simulink model "Quad_F450_Model"  (R2023a)
settings: Solver=FixedStepAuto  StartTime=0.0  StopTime=inf  FixedStep=Copter.SimTs  RelTol=1e-3
InitFcn:
  | load("motor_data.mat")
  | run("Parameters.m")
undefined symbols (not defined in the file or in its folder): Controller, Copter, DiscIntNeverNeededParam, Earth, init, Keyboard, motor_data, w_der_filt, WGS84
libraries: sharedutil x12, slpidlib x8, sharedtransform x5, aerolibpropulsionsys x4, simulink_extras x3, matrix_library x3, shared6dof x1, aerolibtransform2 x1, aerolibatmos2 x1, aerolibsim3d x1, sim3dlib x1
(part 1 of 3)
settings Model: Creator=burak  LastModifiedBy=burak

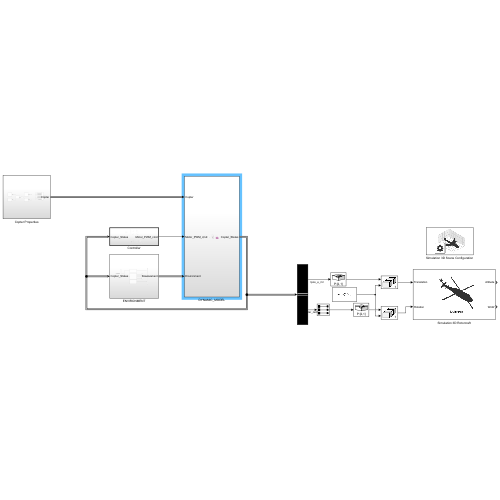
[thumbnail: Simulink's stored preview of the top-level diagram]
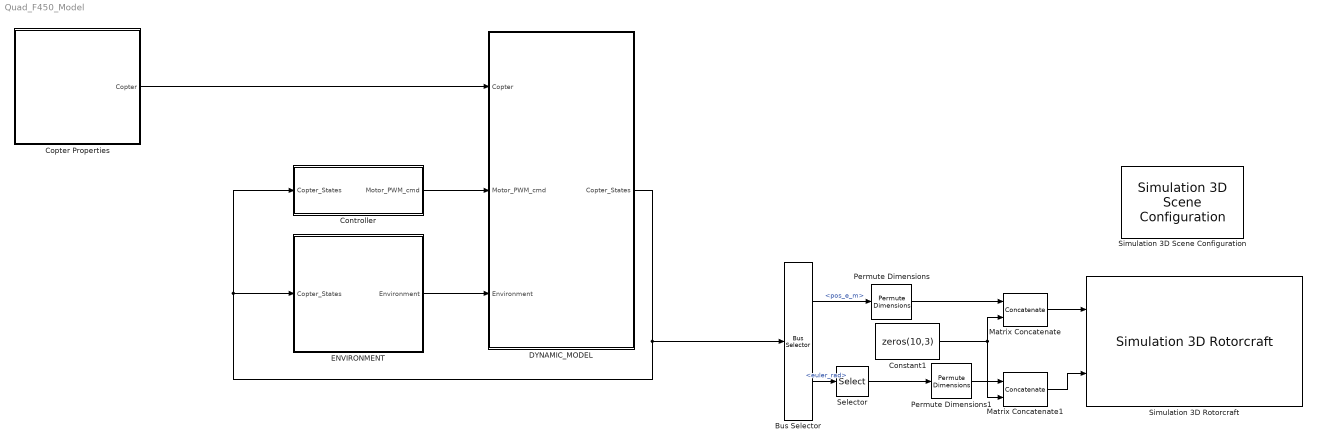
== system Quad_F450_Model ==
  Bus Selector : BusSelector  OutputSignals=pos_e_m,euler_rad
  Constant1 : Constant  Value=zeros(10,3)
  Controller : Subsystem  TreatAsAtomicUnit=on  SystemSampleTime=Controller.Ts
  Copter Properties : Subsystem
  DYNAMIC_MODEL : Subsystem
  ENVIRONMENT : Subsystem
  Matrix Concatenate : Concatenate  Mode=Multidimensional array
  Matrix Concatenate1 : Concatenate  Mode=Multidimensional array
  Permute Dimensions : PermuteDimensions
  Permute Dimensions1 : PermuteDimensions
  Selector : Selector  InputPortWidth=3  IndexOptions=Index vector (dialog)  Indices=[1 2 3]  OutputSizes=1
  Simulation 3D Rotorcraft : aerolibsim3d/Simulation 3D Rotorcraft  Priority=-1  Mesh=Multirotor  MeshPath=/MathWorksAerospaceContent/Vehicles/Rotorcraft/Helicopter/Mesh/SK_Helicopter.SK_Helicopter  MeshPathLight=/MathWorksAerospaceContent/Vehicles/Rotorcraft/LightHelicopter/Mesh/SK_LightHelicopter.SK_LightHelicopter  MeshPathMulti=/MathWorksAerospaceContent/Vehicles/Rotorcraft/Multirotor/Mesh/SK_Quadcopter.SK_Quadcopter  AircraftColor=Red  ActorName=SimulinkVehicle1  Translation=zeros(11, 3)  Rotation=zeros(11, 3)  IsGHSensorEnabled=on  AreGHRaysVisible=off  IsOutputReshapeEnabled=off  GHRayLength=1524  GHBodyOffset=1.169  GHFrontTireRadius=0.196  GHLeftTireRadius=0.203  GHRightTireRadius=0.203  GHContactLocation1=[1.47 -1.04 1.169]  GHContactLocation2=[-1.24 -1.04 1.169]  GHContactLocation3=[-1.24 1.04 1.169]  GHContactLocation4=[1.47 1.04 1.169]  WoWSensorTolerance=0.05  LightsConfig=Automatic lights  LandingLightIntensity=300000  LandingLightConeAngle=15  LandingLightColor=[1 1 1]  HelicopterLeftLandingLightLocation=[0 0 0]  HelicopterLeftLandingLightOrientation=[0 0 0]  NoseLightIntensity=150000  NoseLightConeAngle=36  HelicopterNoseLightLocation=[0 0 0]  HelicopterNoseLightOrientation=[0 0 0]  NavLightIntensity=500  PositionLightIntensity=500  StrobeLightIntensity=5000  StrobeLightColor=[1 1 1]  StrobePeriod=1.5  StrobePulseWidth=6  BeaconLightIntensity=4000  BeaconLightColor=[1 0 0]  BeaconPeriod=1.5  BeaconPulseWidth=10  SampleTime=0.1  ActorType=SimulinkVehicle  ID=1  aMode=0  ActorTag=SimulinkVehicle1
  Simulation 3D Scene Configuration : sim3dlib/Simulation 3D Scene Configuration  Priority=0  ProjectFormat=Unreal Executable  SceneDesc=Airport  ProjectName=C:\Program Files\MATLAB\R2023a\toolbox\shared\sim3d_projects\automotive_project\UE4\WindowsNoEditor\VehicleSimulation.exe  ScenePath=/Game/Maps/HwStrght  EnableOpenDRIVE=off  vehTagList={'Scene Origin';'SimulinkVehicle1'}  vehTag=SimulinkVehicle1  OpVisEn=off  Ts=.02  EnableWindow=on  EnableRemoteAccess=off  EnableWeather=off  SunAltitude=40.0  SunAzimuth=90  clouds=10  wind=1  fog=0  rain=0  EnableGeospatial=off  OriginHeight=200  OriginLatitude=40.744652  OriginLongitude=-73.988864  MapStyle=Aerial  AdditionalAssetIDs=[]  UseAdvancedSunSky=off  SolarTime=11  TimeZone=-5  Day=21  Month=9  Year=2022  UseDaylightSavingTime=on  DSTStartDay=10  DSTStartMonth=3  DSTEndDay=3  DSTEndMonth=11  DSTSwitchHour=2  sensorTag=MainCamera1  sensorId=1  sensorName=MainCamera1  mountLoc=Origin  offsetFlag=off  tmountOffset=[0, 0, 0]  rmountOffset=[0, 0, 0]  HorizontalResolution=1280  VerticalResolution=720  HorizontalFOV=60  mountPoint=[0 0 0]  mountOrientation=[0 0 0]  aMode=0  ID=1  GeoTrigger=Inactive
      settings: LibrarySourceBlock=aerolibsim3d/Simulation 3D Scene Configuration
  wires:
  Copter Properties/1(Copter) -> DYNAMIC_MODEL/1(Copter)
  ENVIRONMENT/1(Environment) -> DYNAMIC_MODEL/3(Environment)
  DYNAMIC_MODEL/1(Copter_States) -> Bus Selector/1, Controller/1(Copter_States), ENVIRONMENT/1(Copter_States)
  Matrix Concatenate/1 -> Simulation 3D Rotorcraft/1
  Bus Selector/1 -> Permute Dimensions/1  "<pos_e_m>"
  Constant1/1 -> Matrix Concatenate1/2, Matrix Concatenate/2
  Permute Dimensions/1 -> Matrix Concatenate/1
  Matrix Concatenate1/1 -> Simulation 3D Rotorcraft/2
  Permute Dimensions1/1 -> Matrix Concatenate1/1
  Bus Selector/2 -> Selector/1  "<euler_rad>"
  Selector/1 -> Permute Dimensions1/1
  Controller/1(Motor_PWM_cmd) -> DYNAMIC_MODEL/2(Motor_PWM_cmd)

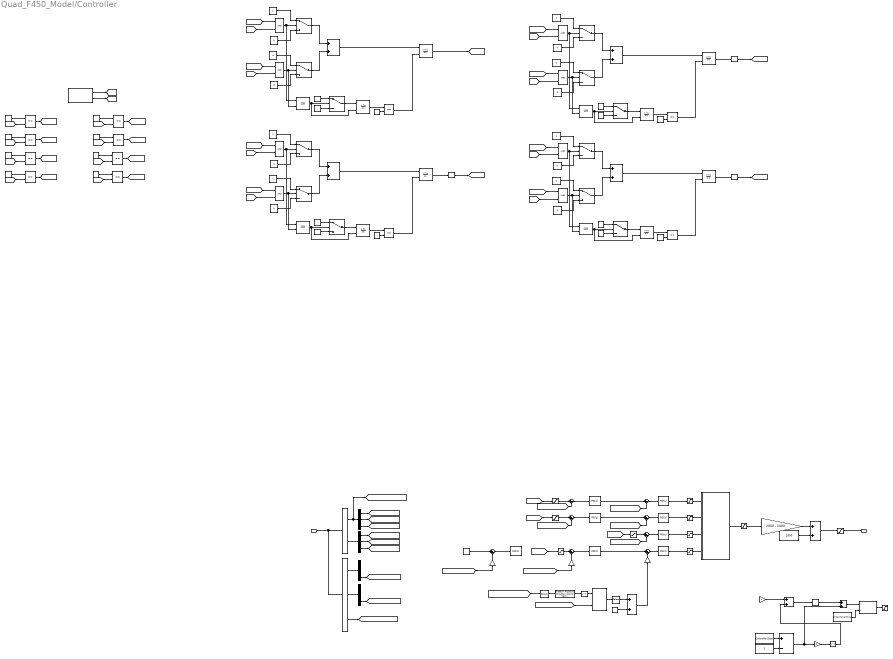
== system Quad_F450_Model/Controller ==
  Copter_States : Inport
  AND{,1..7} (8 alike) : Logic  IconShape=distinctive  AllPortsSameDT=off  OutDataTypeStr=boolean
  Add{,1,3..8} (8 alike) : Sum
  Add2 : Sum  Inputs=+-
  Bus Selector : BusSelector  OutputSignals=euler_rad,angular_vel_b_rads
  Bus Selector1 : BusSelector  OutputSignals=pos_e_m,vel_e_ms,accel_be_mss
  Constant : Constant  Value=9.81
  Constant10 : Constant  Value=30
  Constant11 : Constant  Value=31
  Constant{12..13,15,17..18,21,25..26,28,32..33,35} (12 alike) : Constant  Value=0
  Constant{14,20,27,34} (4 alike) : Constant  Value=-1
  Constant{2..3,6,16,22,24,29,31,36,38} (10 alike) : Constant
  Constant{19,23,30,37} (4 alike) : Constant  Value=Keyboard.Reset
  Constant39 : Constant  Value=101
  Constant4 : Constant  Value=1000
  Constant40 : Constant  Value=113
  Constant41 : Constant  Value=115
  Constant42 : Constant  Value=119
  Constant5 : Constant  Value=Controller.Expo
  Constant7 : Constant  Value=2*Controller.Expo
  Constant8 : Constant  Value=28
  Constant9 : Constant  Value=29
  Degrees to Radians : simulink_extras/Transformations/Degrees to Radians
  Degrees to Radians1 : simulink_extras/Transformations/Degrees to Radians
  Degrees to Radians3 : simulink_extras/Transformations/Degrees to Radians
  Demux{,1..2,4} (4 alike) : Demux  Outputs=3
  Discrete-Time Integrator{,2,4,6} (4 alike) : DiscreteIntegrator  gainval=Keyboard.Gain  ExternalReset=rising  SampleTime=-1  LimitOutput=on  UpperSaturationLimit=20  LowerSaturationLimit=-20  ICPrevOutput=DiscIntNeverNeededParam  ICPrevScaledInput=DiscIntNeverNeededParam
  Discrete-Time Integrator{1,3,5,7} (4 alike) : DiscreteIntegrator  gainval=Keyboard.Reset_Gain  ExternalReset=rising  SampleTime=-1  LimitOutput=on  UpperSaturationLimit=Keyboard.Reset  LowerSaturationLimit=-Keyboard.Reset  ICPrevOutput=DiscIntNeverNeededParam  ICPrevScaledInput=DiscIntNeverNeededParam
  Divide : Product  Inputs=*/
  Equal{,1..11} (12 alike) : RelationalOperator  Operator===  OutDataTypeStr=boolean  RndMeth=Simplest  InputSameDT=off
  Gain{,1..2,5} (4 alike) : Gain  Gain=-1
  Gain3 : Gain  Gain=2000 - 1000
  Gain4 : Gain  Gain=4
  Keyboard 1 : M-S-Function  FunctionName=sfun_keyboard_input_v1_2b  mask(Keyboard Input){}
      mask help: Keyboard Input
      mask Display: fprintf('Keyboard');
  Matrix Multiply : Product  Multiplication=Matrix(*)
  OR{,1..3} (4 alike) : Logic  Operator=OR  IconShape=distinctive  AllPortsSameDT=off  OutDataTypeStr=boolean
  PID Controller : slpidlib/PID Controller  Controller=PID  Form=Parallel  TimeDomain=Discrete-time  UseExternalTs=off  SampleTime=Controller.Ts  IntegratorMethod=Forward Euler  FilterMethod=Forward Euler  ControllerParametersSource=internal  P=1  I=1  UseKiTs=off  D=1/37.5  N=2*pi*20  UseFilter=on  TunerSelectOption=Transfer Function Based (PID Tuner App)  InitialConditionSource=internal  InitialConditionForIntegrator=0  InitialConditionForFilter=0  DifferentiatorICPrevScaledInput=0  ExternalReset=none  TrackingMode=off  Kt=1  LimitOutput=on  SatLimitsSource=internal  UpperSaturationLimit=1  LowerSaturationLimit=-1  LinearizeAsGain=on  AntiWindupMode=clamping  Kb=1  LimitIntegrator=on  UpperIntegratorSaturationLimit=1  LowerIntegratorSaturationLimit=-1  POutMin=[]  POutMax=[]  IOutMin=[]  IOutMax=[]  DOutMin=[]  DOutMax=[]  NOutMin=[]  NOutMax=[]  SumOutMin=[]  SumOutMax=[]  SaturationOutMin=[]  SaturationOutMax=[]  PParamMin=[]  PParamMax=[]  IParamMin=[]  IParamMax=[]  DParamMin=[]  DParamMax=[]  NParamMin=[]  NParamMax=[]  KbParamMin=[]  KbParamMax=[]  KtParamMin=[]  KtParamMax=[]  KbOutMin=[]  KbOutMax=[]  KtOutMin=[]  KtOutMax=[]  IntegratorOutMin=[]  IntegratorOutMax=[]  FilterOutMin=[]  FilterOutMax=[]  SumI1OutMin=[]  SumI1OutMax=[]  SumI2OutMin=[]  SumI2OutMax=[]  SumI3OutMin=[]  SumI3OutMax=[]  SumI4OutMin=[]  SumI4OutMax=[]  SumDOutMin=[]  SumDOutMax=[]  DifferentiatorOutMin=[]  DifferentiatorOutMax=[]  FilterDiffOutCoefMin=[]  FilterDiffOutCoefMax=[]  ReciprocalOutMin=[]  ReciprocalOutMax=[]  SumDenOutMin=[]  SumDenOutMax=[]  SumNumOutMin=[]  SumNumOutMax=[]  DivideOutMin=[]  DivideOutMax=[]  UdiffTsProdOutMin=[]  UdiffTsProdOutMax=[]  NTsProdOutMin=[]  NTsProdOutMax=[]  UintegralTsProdOutMin=[]  UintegralTsProdOutMax=[]  UngainTsProdOutMin=[]  UngainTsProdOutMax=[]  ClampingZeroOutDataTypeStr=Inherit: Inherit via back propagation  ClampingZeroOutMin=[]  ClampingZeroOutMax=[]  FilterDenConstantOutDataTypeStr=Inherit: Inherit via back propagation  FilterDenConstantOutMin=[]  FilterDenConstantOutMax=[]  PCopyOutDataTypeStr=Inherit: Inherit via back propagation  PCopyOutMin=[]  PCopyOutMax=[]  NCopyOutDataTypeStr=Inherit: Inherit via back propagation  NCopyOutMin=[]  NCopyOutMax=[]  IntegratorContinuousStateAttributes=''  IntegratorStateMustResolveToSignalObject=off  IntegratorRTWStateStorageClass=Auto  FilterContinuousStateAttributes=''  FilterStateMustResolveToSignalObject=off  FilterRTWStateStorageClass=Auto  ParallelPVariant=InternalParameters  IdealPVariant=Disabled  IVariant=InternalParameters  DVariant=InternalParameters  IntegratorVariant=Discrete  SatVariant=Enabled  AWVariant=DiscClampingParallel  PCopyVariant=Disabled  TRVariant=Disabled  FdbkBlocksVariant=Forward  IdealPFdbkVariant=Disabled  SatFdbkVariant=Disabled  DerivativeFilterVariant=ForwardEulerFilter  NVariant=InternalParameters  NCopyVariant=Disabled  FilterICVariant=InternalICsFilter  IntegratorICVariant=InternalICs  ExternalResetVariant=Disabled  TRSumVariant=Passthrough  SumFdbkVariant=Disabled  SumVariant=Sum_PID  TsampFilterVariant=InternalTs  TsampNgainVariant=Passthrough  TsampIntegralVariant=Disabled_SignalSpec  ExternalSaturationOutDataTypeStr=Inherit: Same as second input
  PID Controller1 : slpidlib/PID Controller  Controller=PID  Form=Parallel  TimeDomain=Discrete-time  UseExternalTs=off  SampleTime=Controller.Ts  IntegratorMethod=Forward Euler  FilterMethod=Forward Euler  ControllerParametersSource=internal  P=1  I=1  UseKiTs=off  D=1/37.5  N=2*pi*20  UseFilter=on  TunerSelectOption=Transfer Function Based (PID Tuner App)  InitialConditionSource=internal  InitialConditionForIntegrator=0  InitialConditionForFilter=0  DifferentiatorICPrevScaledInput=0  ExternalReset=none  TrackingMode=off  Kt=1  LimitOutput=on  SatLimitsSource=internal  UpperSaturationLimit=1  LowerSaturationLimit=-1  LinearizeAsGain=on  AntiWindupMode=clamping  Kb=1  LimitIntegrator=on  UpperIntegratorSaturationLimit=1  LowerIntegratorSaturationLimit=-1  POutMin=[]  POutMax=[]  IOutMin=[]  IOutMax=[]  DOutMin=[]  DOutMax=[]  NOutMin=[]  NOutMax=[]  SumOutMin=[]  SumOutMax=[]  SaturationOutMin=[]  SaturationOutMax=[]  PParamMin=[]  PParamMax=[]  IParamMin=[]  IParamMax=[]  DParamMin=[]  DParamMax=[]  NParamMin=[]  NParamMax=[]  KbParamMin=[]  KbParamMax=[]  KtParamMin=[]  KtParamMax=[]  KbOutMin=[]  KbOutMax=[]  KtOutMin=[]  KtOutMax=[]  IntegratorOutMin=[]  IntegratorOutMax=[]  FilterOutMin=[]  FilterOutMax=[]  SumI1OutMin=[]  SumI1OutMax=[]  SumI2OutMin=[]  SumI2OutMax=[]  SumI3OutMin=[]  SumI3OutMax=[]  SumI4OutMin=[]  SumI4OutMax=[]  SumDOutMin=[]  SumDOutMax=[]  DifferentiatorOutMin=[]  DifferentiatorOutMax=[]  FilterDiffOutCoefMin=[]  FilterDiffOutCoefMax=[]  ReciprocalOutMin=[]  ReciprocalOutMax=[]  SumDenOutMin=[]  SumDenOutMax=[]  SumNumOutMin=[]  SumNumOutMax=[]  DivideOutMin=[]  DivideOutMax=[]  UdiffTsProdOutMin=[]  UdiffTsProdOutMax=[]  NTsProdOutMin=[]  NTsProdOutMax=[]  UintegralTsProdOutMin=[]  UintegralTsProdOutMax=[]  UngainTsProdOutMin=[]  UngainTsProdOutMax=[]  ClampingZeroOutDataTypeStr=Inherit: Inherit via back propagation  ClampingZeroOutMin=[]  ClampingZeroOutMax=[]  FilterDenConstantOutDataTypeStr=Inherit: Inherit via back propagation  FilterDenConstantOutMin=[]  FilterDenConstantOutMax=[]  PCopyOutDataTypeStr=Inherit: Inherit via back propagation  PCopyOutMin=[]  PCopyOutMax=[]  NCopyOutDataTypeStr=Inherit: Inherit via back propagation  NCopyOutMin=[]  NCopyOutMax=[]  IntegratorContinuousStateAttributes=''  IntegratorStateMustResolveToSignalObject=off  IntegratorRTWStateStorageClass=Auto  FilterContinuousStateAttributes=''  FilterStateMustResolveToSignalObject=off  FilterRTWStateStorageClass=Auto  ParallelPVariant=InternalParameters  IdealPVariant=Disabled  IVariant=InternalParameters  DVariant=InternalParameters  IntegratorVariant=Discrete  SatVariant=Enabled  AWVariant=DiscClampingParallel  PCopyVariant=Disabled  TRVariant=Disabled  FdbkBlocksVariant=Forward  IdealPFdbkVariant=Disabled  SatFdbkVariant=Disabled  DerivativeFilterVariant=ForwardEulerFilter  NVariant=InternalParameters  NCopyVariant=Disabled  FilterICVariant=InternalICsFilter  IntegratorICVariant=InternalICs  ExternalResetVariant=Disabled  TRSumVariant=Passthrough  SumFdbkVariant=Disabled  SumVariant=Sum_PID  TsampFilterVariant=InternalTs  TsampNgainVariant=Passthrough  TsampIntegralVariant=Disabled_SignalSpec  ExternalSaturationOutDataTypeStr=Inherit: Same as second input
  PID Controller2 : slpidlib/PID Controller  Controller=PID  Form=Parallel  TimeDomain=Discrete-time  UseExternalTs=off  SampleTime=Controller.Ts  IntegratorMethod=Forward Euler  FilterMethod=Forward Euler  ControllerParametersSource=internal  P=1  I=1  UseKiTs=off  D=0  N=2*pi*20  UseFilter=on  TunerSelectOption=Transfer Function Based (PID Tuner App)  InitialConditionSource=internal  InitialConditionForIntegrator=0  InitialConditionForFilter=0  DifferentiatorICPrevScaledInput=0  ExternalReset=none  TrackingMode=off  Kt=1  LimitOutput=on  SatLimitsSource=internal  UpperSaturationLimit=1  LowerSaturationLimit=-1  LinearizeAsGain=on  AntiWindupMode=clamping  Kb=1  LimitIntegrator=on  UpperIntegratorSaturationLimit=1  LowerIntegratorSaturationLimit=-1  POutMin=[]  POutMax=[]  IOutMin=[]  IOutMax=[]  DOutMin=[]  DOutMax=[]  NOutMin=[]  NOutMax=[]  SumOutMin=[]  SumOutMax=[]  SaturationOutMin=[]  SaturationOutMax=[]  PParamMin=[]  PParamMax=[]  IParamMin=[]  IParamMax=[]  DParamMin=[]  DParamMax=[]  NParamMin=[]  NParamMax=[]  KbParamMin=[]  KbParamMax=[]  KtParamMin=[]  KtParamMax=[]  KbOutMin=[]  KbOutMax=[]  KtOutMin=[]  KtOutMax=[]  IntegratorOutMin=[]  IntegratorOutMax=[]  FilterOutMin=[]  FilterOutMax=[]  SumI1OutMin=[]  SumI1OutMax=[]  SumI2OutMin=[]  SumI2OutMax=[]  SumI3OutMin=[]  SumI3OutMax=[]  SumI4OutMin=[]  SumI4OutMax=[]  SumDOutMin=[]  SumDOutMax=[]  DifferentiatorOutMin=[]  DifferentiatorOutMax=[]  FilterDiffOutCoefMin=[]  FilterDiffOutCoefMax=[]  ReciprocalOutMin=[]  ReciprocalOutMax=[]  SumDenOutMin=[]  SumDenOutMax=[]  SumNumOutMin=[]  SumNumOutMax=[]  DivideOutMin=[]  DivideOutMax=[]  UdiffTsProdOutMin=[]  UdiffTsProdOutMax=[]  NTsProdOutMin=[]  NTsProdOutMax=[]  UintegralTsProdOutMin=[]  UintegralTsProdOutMax=[]  UngainTsProdOutMin=[]  UngainTsProdOutMax=[]  ClampingZeroOutDataTypeStr=Inherit: Inherit via back propagation  ClampingZeroOutMin=[]  ClampingZeroOutMax=[]  FilterDenConstantOutDataTypeStr=Inherit: Inherit via back propagation  FilterDenConstantOutMin=[]  FilterDenConstantOutMax=[]  PCopyOutDataTypeStr=Inherit: Inherit via back propagation  PCopyOutMin=[]  PCopyOutMax=[]  NCopyOutDataTypeStr=Inherit: Inherit via back propagation  NCopyOutMin=[]  NCopyOutMax=[]  IntegratorContinuousStateAttributes=''  IntegratorStateMustResolveToSignalObject=off  IntegratorRTWStateStorageClass=Auto  FilterContinuousStateAttributes=''  FilterStateMustResolveToSignalObject=off  FilterRTWStateStorageClass=Auto  ParallelPVariant=InternalParameters  IdealPVariant=Disabled  IVariant=InternalParameters  DVariant=InternalParameters  IntegratorVariant=Discrete  SatVariant=Enabled  AWVariant=DiscClampingParallel  PCopyVariant=Disabled  TRVariant=Disabled  FdbkBlocksVariant=Forward  IdealPFdbkVariant=Disabled  SatFdbkVariant=Disabled  DerivativeFilterVariant=ForwardEulerFilter  NVariant=InternalParameters  NCopyVariant=Disabled  FilterICVariant=InternalICsFilter  IntegratorICVariant=InternalICs  ExternalResetVariant=Disabled  TRSumVariant=Passthrough  SumFdbkVariant=Disabled  SumVariant=Sum_PID  TsampFilterVariant=InternalTs  TsampNgainVariant=Passthrough  TsampIntegralVariant=Disabled_SignalSpec  ExternalSaturationOutDataTypeStr=Inherit: Same as second input
  PID Controller3 : slpidlib/PID Controller  Controller=PID  Form=Parallel  TimeDomain=Discrete-time  UseExternalTs=off  SampleTime=Controller.Ts  IntegratorMethod=Forward Euler  FilterMethod=Forward Euler  ControllerParametersSource=internal  P=4.5  I=0  UseKiTs=off  D=0  N=100  UseFilter=on  TunerSelectOption=Transfer Function Based (PID Tuner App)  InitialConditionSource=internal  InitialConditionForIntegrator=0  InitialConditionForFilter=0  DifferentiatorICPrevScaledInput=0  ExternalReset=none  TrackingMode=off  Kt=1  LimitOutput=on  SatLimitsSource=internal  UpperSaturationLimit=deg2rad(200)  LowerSaturationLimit=-deg2rad(200)  LinearizeAsGain=on  AntiWindupMode=clamping  Kb=1  LimitIntegrator=on  UpperIntegratorSaturationLimit=deg2rad(200)  LowerIntegratorSaturationLimit=-deg2rad(200)  POutMin=[]  POutMax=[]  IOutMin=[]  IOutMax=[]  DOutMin=[]  DOutMax=[]  NOutMin=[]  NOutMax=[]  SumOutMin=[]  SumOutMax=[]  SaturationOutMin=[]  SaturationOutMax=[]  PParamMin=[]  PParamMax=[]  IParamMin=[]  IParamMax=[]  DParamMin=[]  DParamMax=[]  NParamMin=[]  NParamMax=[]  KbParamMin=[]  KbParamMax=[]  KtParamMin=[]  KtParamMax=[]  KbOutMin=[]  KbOutMax=[]  KtOutMin=[]  KtOutMax=[]  IntegratorOutMin=[]  IntegratorOutMax=[]  FilterOutMin=[]  FilterOutMax=[]  SumI1OutMin=[]  SumI1OutMax=[]  SumI2OutMin=[]  SumI2OutMax=[]  SumI3OutMin=[]  SumI3OutMax=[]  SumI4OutMin=[]  SumI4OutMax=[]  SumDOutMin=[]  SumDOutMax=[]  DifferentiatorOutMin=[]  DifferentiatorOutMax=[]  FilterDiffOutCoefMin=[]  FilterDiffOutCoefMax=[]  ReciprocalOutMin=[]  ReciprocalOutMax=[]  SumDenOutMin=[]  SumDenOutMax=[]  SumNumOutMin=[]  SumNumOutMax=[]  DivideOutMin=[]  DivideOutMax=[]  UdiffTsProdOutMin=[]  UdiffTsProdOutMax=[]  NTsProdOutMin=[]  NTsProdOutMax=[]  UintegralTsProdOutMin=[]  UintegralTsProdOutMax=[]  UngainTsProdOutMin=[]  UngainTsProdOutMax=[]  ClampingZeroOutDataTypeStr=Inherit: Inherit via back propagation  ClampingZeroOutMin=[]  ClampingZeroOutMax=[]  FilterDenConstantOutDataTypeStr=Inherit: Inherit via back propagation  FilterDenConstantOutMin=[]  FilterDenConstantOutMax=[]  PCopyOutDataTypeStr=Inherit: Inherit via back propagation  PCopyOutMin=[]  PCopyOutMax=[]  NCopyOutDataTypeStr=Inherit: Inherit via back propagation  NCopyOutMin=[]  NCopyOutMax=[]  IntegratorContinuousStateAttributes=''  IntegratorStateMustResolveToSignalObject=off  IntegratorRTWStateStorageClass=Auto  FilterContinuousStateAttributes=''  FilterStateMustResolveToSignalObject=off  FilterRTWStateStorageClass=Auto  ParallelPVariant=InternalParameters  IdealPVariant=Disabled  IVariant=InternalParameters  DVariant=InternalParameters  IntegratorVariant=Discrete  SatVariant=Enabled  AWVariant=DiscClampingParallel  PCopyVariant=Disabled  TRVariant=Disabled  FdbkBlocksVariant=Forward  IdealPFdbkVariant=Disabled  SatFdbkVariant=Disabled  DerivativeFilterVariant=ForwardEulerFilter  NVariant=InternalParameters  NCopyVariant=Disabled  FilterICVariant=InternalICsFilter  IntegratorICVariant=InternalICs  ExternalResetVariant=Disabled  TRSumVariant=Passthrough  SumFdbkVariant=Disabled  SumVariant=Sum_PID  TsampFilterVariant=InternalTs  TsampNgainVariant=Passthrough  TsampIntegralVariant=Disabled_SignalSpec  ExternalSaturationOutDataTypeStr=Inherit: Same as second input
  PID Controller4 : slpidlib/PID Controller  Controller=PID  Form=Parallel  TimeDomain=Discrete-time  UseExternalTs=off  SampleTime=Controller.Ts  IntegratorMethod=Forward Euler  FilterMethod=Forward Euler  ControllerParametersSource=internal  P=4.5  I=0  UseKiTs=off  D=0  N=100  UseFilter=on  TunerSelectOption=Transfer Function Based (PID Tuner App)  InitialConditionSource=internal  InitialConditionForIntegrator=0  InitialConditionForFilter=0  DifferentiatorICPrevScaledInput=0  ExternalReset=none  TrackingMode=off  Kt=1  LimitOutput=on  SatLimitsSource=internal  UpperSaturationLimit=deg2rad(200)  LowerSaturationLimit=-deg2rad(200)  LinearizeAsGain=on  AntiWindupMode=clamping  Kb=1  LimitIntegrator=on  UpperIntegratorSaturationLimit=deg2rad(200)  LowerIntegratorSaturationLimit=-deg2rad(200)  POutMin=[]  POutMax=[]  IOutMin=[]  IOutMax=[]  DOutMin=[]  DOutMax=[]  NOutMin=[]  NOutMax=[]  SumOutMin=[]  SumOutMax=[]  SaturationOutMin=[]  SaturationOutMax=[]  PParamMin=[]  PParamMax=[]  IParamMin=[]  IParamMax=[]  DParamMin=[]  DParamMax=[]  NParamMin=[]  NParamMax=[]  KbParamMin=[]  KbParamMax=[]  KtParamMin=[]  KtParamMax=[]  KbOutMin=[]  KbOutMax=[]  KtOutMin=[]  KtOutMax=[]  IntegratorOutMin=[]  IntegratorOutMax=[]  FilterOutMin=[]  FilterOutMax=[]  SumI1OutMin=[]  SumI1OutMax=[]  SumI2OutMin=[]  SumI2OutMax=[]  SumI3OutMin=[]  SumI3OutMax=[]  SumI4OutMin=[]  SumI4OutMax=[]  SumDOutMin=[]  SumDOutMax=[]  DifferentiatorOutMin=[]  DifferentiatorOutMax=[]  FilterDiffOutCoefMin=[]  FilterDiffOutCoefMax=[]  ReciprocalOutMin=[]  ReciprocalOutMax=[]  SumDenOutMin=[]  SumDenOutMax=[]  SumNumOutMin=[]  SumNumOutMax=[]  DivideOutMin=[]  DivideOutMax=[]  UdiffTsProdOutMin=[]  UdiffTsProdOutMax=[]  NTsProdOutMin=[]  NTsProdOutMax=[]  UintegralTsProdOutMin=[]  UintegralTsProdOutMax=[]  UngainTsProdOutMin=[]  UngainTsProdOutMax=[]  ClampingZeroOutDataTypeStr=Inherit: Inherit via back propagation  ClampingZeroOutMin=[]  ClampingZeroOutMax=[]  FilterDenConstantOutDataTypeStr=Inherit: Inherit via back propagation  FilterDenConstantOutMin=[]  FilterDenConstantOutMax=[]  PCopyOutDataTypeStr=Inherit: Inherit via back propagation  PCopyOutMin=[]  PCopyOutMax=[]  NCopyOutDataTypeStr=Inherit: Inherit via back propagation  NCopyOutMin=[]  NCopyOutMax=[]  IntegratorContinuousStateAttributes=''  IntegratorStateMustResolveToSignalObject=off  IntegratorRTWStateStorageClass=Auto  FilterContinuousStateAttributes=''  FilterStateMustResolveToSignalObject=off  FilterRTWStateStorageClass=Auto  ParallelPVariant=InternalParameters  IdealPVariant=Disabled  IVariant=InternalParameters  DVariant=InternalParameters  IntegratorVariant=Discrete  SatVariant=Enabled  AWVariant=DiscClampingParallel  PCopyVariant=Disabled  TRVariant=Disabled  FdbkBlocksVariant=Forward  IdealPFdbkVariant=Disabled  SatFdbkVariant=Disabled  DerivativeFilterVariant=ForwardEulerFilter  NVariant=InternalParameters  NCopyVariant=Disabled  FilterICVariant=InternalICsFilter  IntegratorICVariant=InternalICs  ExternalResetVariant=Disabled  TRSumVariant=Passthrough  SumFdbkVariant=Disabled  SumVariant=Sum_PID  TsampFilterVariant=InternalTs  TsampNgainVariant=Passthrough  TsampIntegralVariant=Disabled_SignalSpec  ExternalSaturationOutDataTypeStr=Inherit: Same as second input
  PID Controller5 : slpidlib/PID Controller  Controller=PID  Form=Parallel  TimeDomain=Discrete-time  UseExternalTs=off  SampleTime=Controller.Ts  IntegratorMethod=Forward Euler  FilterMethod=Forward Euler  ControllerParametersSource=internal  P=0.5  I=1  UseKiTs=off  D=0  N=100  UseFilter=on  TunerSelectOption=Transfer Function Based (PID Tuner App)  InitialConditionSource=internal  InitialConditionForIntegrator=0  InitialConditionForFilter=0  DifferentiatorICPrevScaledInput=0  ExternalReset=none  TrackingMode=off  Kt=1  LimitOutput=on  SatLimitsSource=internal  UpperSaturationLimit=1  LowerSaturationLimit=-1  LinearizeAsGain=on  AntiWindupMode=clamping  Kb=1  LimitIntegrator=on  UpperIntegratorSaturationLimit=1  LowerIntegratorSaturationLimit=-1  POutMin=[]  POutMax=[]  IOutMin=[]  IOutMax=[]  DOutMin=[]  DOutMax=[]  NOutMin=[]  NOutMax=[]  SumOutMin=[]  SumOutMax=[]  SaturationOutMin=[]  SaturationOutMax=[]  PParamMin=[]  PParamMax=[]  IParamMin=[]  IParamMax=[]  DParamMin=[]  DParamMax=[]  NParamMin=[]  NParamMax=[]  KbParamMin=[]  KbParamMax=[]  KtParamMin=[]  KtParamMax=[]  KbOutMin=[]  KbOutMax=[]  KtOutMin=[]  KtOutMax=[]  IntegratorOutMin=[]  IntegratorOutMax=[]  FilterOutMin=[]  FilterOutMax=[]  SumI1OutMin=[]  SumI1OutMax=[]  SumI2OutMin=[]  SumI2OutMax=[]  SumI3OutMin=[]  SumI3OutMax=[]  SumI4OutMin=[]  SumI4OutMax=[]  SumDOutMin=[]  SumDOutMax=[]  DifferentiatorOutMin=[]  DifferentiatorOutMax=[]  FilterDiffOutCoefMin=[]  FilterDiffOutCoefMax=[]  ReciprocalOutMin=[]  ReciprocalOutMax=[]  SumDenOutMin=[]  SumDenOutMax=[]  SumNumOutMin=[]  SumNumOutMax=[]  DivideOutMin=[]  DivideOutMax=[]  UdiffTsProdOutMin=[]  UdiffTsProdOutMax=[]  NTsProdOutMin=[]  NTsProdOutMax=[]  UintegralTsProdOutMin=[]  UintegralTsProdOutMax=[]  UngainTsProdOutMin=[]  UngainTsProdOutMax=[]  ClampingZeroOutDataTypeStr=Inherit: Inherit via back propagation  ClampingZeroOutMin=[]  ClampingZeroOutMax=[]  FilterDenConstantOutDataTypeStr=Inherit: Inherit via back propagation  FilterDenConstantOutMin=[]  FilterDenConstantOutMax=[]  PCopyOutDataTypeStr=Inherit: Inherit via back propagation  PCopyOutMin=[]  PCopyOutMax=[]  NCopyOutDataTypeStr=Inherit: Inherit via back propagation  NCopyOutMin=[]  NCopyOutMax=[]  IntegratorContinuousStateAttributes=''  IntegratorStateMustResolveToSignalObject=off  IntegratorRTWStateStorageClass=Auto  FilterContinuousStateAttributes=''  FilterStateMustResolveToSignalObject=off  FilterRTWStateStorageClass=Auto  ParallelPVariant=InternalParameters  IdealPVariant=Disabled  IVariant=InternalParameters  DVariant=InternalParameters  IntegratorVariant=Discrete  SatVariant=Enabled  AWVariant=DiscClampingParallel  PCopyVariant=Disabled  TRVariant=Disabled  FdbkBlocksVariant=Forward  IdealPFdbkVariant=Disabled  SatFdbkVariant=Disabled  DerivativeFilterVariant=ForwardEulerFilter  NVariant=InternalParameters  NCopyVariant=Disabled  FilterICVariant=InternalICsFilter  IntegratorICVariant=InternalICs  ExternalResetVariant=Disabled  TRSumVariant=Passthrough  SumFdbkVariant=Disabled  SumVariant=Sum_PID  TsampFilterVariant=InternalTs  TsampNgainVariant=Passthrough  TsampIntegralVariant=Disabled_SignalSpec  ExternalSaturationOutDataTypeStr=Inherit: Same as second input
  PID Controller6 : slpidlib/PID Controller  Controller=PID  Form=Parallel  TimeDomain=Discrete-time  UseExternalTs=off  SampleTime=Controller.Ts  IntegratorMethod=Forward Euler  FilterMethod=Forward Euler  ControllerParametersSource=internal  P=5  I=5  UseKiTs=off  D=0  N=100  UseFilter=on  TunerSelectOption=Transfer Function Based (PID Tuner App)  InitialConditionSource=internal  InitialConditionForIntegrator=0  InitialConditionForFilter=0  DifferentiatorICPrevScaledInput=0  ExternalReset=none  TrackingMode=off  Kt=1  LimitOutput=off  SatLimitsSource=internal  UpperSaturationLimit=5  LowerSaturationLimit=-5  LinearizeAsGain=on  AntiWindupMode=none  Kb=1  LimitIntegrator=off  UpperIntegratorSaturationLimit=10  LowerIntegratorSaturationLimit=-10  POutMin=[]  POutMax=[]  IOutMin=[]  IOutMax=[]  DOutMin=[]  DOutMax=[]  NOutMin=[]  NOutMax=[]  SumOutMin=[]  SumOutMax=[]  SaturationOutMin=[]  SaturationOutMax=[]  PParamMin=[]  PParamMax=[]  IParamMin=[]  IParamMax=[]  DParamMin=[]  DParamMax=[]  NParamMin=[]  NParamMax=[]  KbParamMin=[]  KbParamMax=[]  KtParamMin=[]  KtParamMax=[]  KbOutMin=[]  KbOutMax=[]  KtOutMin=[]  KtOutMax=[]  IntegratorOutMin=[]  IntegratorOutMax=[]  FilterOutMin=[]  FilterOutMax=[]  SumI1OutMin=[]  SumI1OutMax=[]  SumI2OutMin=[]  SumI2OutMax=[]  SumI3OutMin=[]  SumI3OutMax=[]  SumI4OutMin=[]  SumI4OutMax=[]  SumDOutMin=[]  SumDOutMax=[]  DifferentiatorOutMin=[]  DifferentiatorOutMax=[]  FilterDiffOutCoefMin=[]  FilterDiffOutCoefMax=[]  ReciprocalOutMin=[]  ReciprocalOutMax=[]  SumDenOutMin=[]  SumDenOutMax=[]  SumNumOutMin=[]  SumNumOutMax=[]  DivideOutMin=[]  DivideOutMax=[]  UdiffTsProdOutMin=[]  UdiffTsProdOutMax=[]  NTsProdOutMin=[]  NTsProdOutMax=[]  UintegralTsProdOutMin=[]  UintegralTsProdOutMax=[]  UngainTsProdOutMin=[]  UngainTsProdOutMax=[]  ClampingZeroOutDataTypeStr=Inherit: Inherit via back propagation  ClampingZeroOutMin=[]  ClampingZeroOutMax=[]  FilterDenConstantOutDataTypeStr=Inherit: Inherit via back propagation  FilterDenConstantOutMin=[]  FilterDenConstantOutMax=[]  PCopyOutDataTypeStr=Inherit: Inherit via back propagation  PCopyOutMin=[]  PCopyOutMax=[]  NCopyOutDataTypeStr=Inherit: Inherit via back propagation  NCopyOutMin=[]  NCopyOutMax=[]  IntegratorContinuousStateAttributes=''  IntegratorStateMustResolveToSignalObject=off  IntegratorRTWStateStorageClass=Auto  FilterContinuousStateAttributes=''  FilterStateMustResolveToSignalObject=off  FilterRTWStateStorageClass=Auto  ParallelPVariant=InternalParameters  IdealPVariant=Disabled  IVariant=InternalParameters  DVariant=InternalParameters  IntegratorVariant=Discrete  SatVariant=Disabled  AWVariant=Passthrough  PCopyVariant=Disabled  TRVariant=Disabled  FdbkBlocksVariant=Forward  IdealPFdbkVariant=Disabled  SatFdbkVariant=Disabled  DerivativeFilterVariant=ForwardEulerFilter  NVariant=InternalParameters  NCopyVariant=Disabled  FilterICVariant=InternalICsFilter  IntegratorICVariant=InternalICs  ExternalResetVariant=Disabled  TRSumVariant=Passthrough  SumFdbkVariant=Disabled  SumVariant=Sum_PID  TsampFilterVariant=InternalTs  TsampNgainVariant=Passthrough  TsampIntegralVariant=Disabled_SignalSpec  ExternalSaturationOutDataTypeStr=Inherit: Same as second input
  PID Controller7 : slpidlib/PID Controller  Controller=PID  Form=Parallel  TimeDomain=Discrete-time  UseExternalTs=off  SampleTime=Controller.Ts  IntegratorMethod=Forward Euler  FilterMethod=Forward Euler  ControllerParametersSource=internal  P=1  I=0  UseKiTs=off  D=0  N=100  UseFilter=on  TunerSelectOption=Transfer Function Based (PID Tuner App)  InitialConditionSource=internal  InitialConditionForIntegrator=0  InitialConditionForFilter=0  DifferentiatorICPrevScaledInput=0  ExternalReset=none  TrackingMode=off  Kt=1  LimitOutput=off  SatLimitsSource=internal  UpperSaturationLimit=inf  LowerSaturationLimit=-inf  LinearizeAsGain=on  AntiWindupMode=none  Kb=1  LimitIntegrator=off  UpperIntegratorSaturationLimit=inf  LowerIntegratorSaturationLimit=-inf  POutMin=[]  POutMax=[]  IOutMin=[]  IOutMax=[]  DOutMin=[]  DOutMax=[]  NOutMin=[]  NOutMax=[]  SumOutMin=[]  SumOutMax=[]  SaturationOutMin=[]  SaturationOutMax=[]  PParamMin=[]  PParamMax=[]  IParamMin=[]  IParamMax=[]  DParamMin=[]  DParamMax=[]  NParamMin=[]  NParamMax=[]  KbParamMin=[]  KbParamMax=[]  KtParamMin=[]  KtParamMax=[]  KbOutMin=[]  KbOutMax=[]  KtOutMin=[]  KtOutMax=[]  IntegratorOutMin=[]  IntegratorOutMax=[]  FilterOutMin=[]  FilterOutMax=[]  SumI1OutMin=[]  SumI1OutMax=[]  SumI2OutMin=[]  SumI2OutMax=[]  SumI3OutMin=[]  SumI3OutMax=[]  SumI4OutMin=[]  SumI4OutMax=[]  SumDOutMin=[]  SumDOutMax=[]  DifferentiatorOutMin=[]  DifferentiatorOutMax=[]  FilterDiffOutCoefMin=[]  FilterDiffOutCoefMax=[]  ReciprocalOutMin=[]  ReciprocalOutMax=[]  SumDenOutMin=[]  SumDenOutMax=[]  SumNumOutMin=[]  SumNumOutMax=[]  DivideOutMin=[]  DivideOutMax=[]  UdiffTsProdOutMin=[]  UdiffTsProdOutMax=[]  NTsProdOutMin=[]  NTsProdOutMax=[]  UintegralTsProdOutMin=[]  UintegralTsProdOutMax=[]  UngainTsProdOutMin=[]  UngainTsProdOutMax=[]  ClampingZeroOutDataTypeStr=Inherit: Inherit via back propagation  ClampingZeroOutMin=[]  ClampingZeroOutMax=[]  FilterDenConstantOutDataTypeStr=Inherit: Inherit via back propagation  FilterDenConstantOutMin=[]  FilterDenConstantOutMax=[]  PCopyOutDataTypeStr=Inherit: Inherit via back propagation  PCopyOutMin=[]  PCopyOutMax=[]  NCopyOutDataTypeStr=Inherit: Inherit via back propagation  NCopyOutMin=[]  NCopyOutMax=[]  IntegratorContinuousStateAttributes=''  IntegratorStateMustResolveToSignalObject=off  IntegratorRTWStateStorageClass=Auto  FilterContinuousStateAttributes=''  FilterStateMustResolveToSignalObject=off  FilterRTWStateStorageClass=Auto  ParallelPVariant=InternalParameters  IdealPVariant=Disabled  IVariant=InternalParameters  DVariant=InternalParameters  IntegratorVariant=Discrete  SatVariant=Disabled  AWVariant=Passthrough  PCopyVariant=Disabled  TRVariant=Disabled  FdbkBlocksVariant=Forward  IdealPFdbkVariant=Disabled  SatFdbkVariant=Disabled  DerivativeFilterVariant=ForwardEulerFilter  NVariant=InternalParameters  NCopyVariant=Disabled  FilterICVariant=InternalICsFilter  IntegratorICVariant=InternalICs  ExternalResetVariant=Disabled  TRSumVariant=Passthrough  SumFdbkVariant=Disabled  SumVariant=Sum_PID  TsampFilterVariant=InternalTs  TsampNgainVariant=Passthrough  TsampIntegralVariant=Disabled_SignalSpec  ExternalSaturationOutDataTypeStr=Inherit: Same as second input
  Rotation Angles to Direction Cosine Matrix : sharedtransform/Rotation Angles to Direction Cosine Matrix  rotationOrder=ZYX  aMode=aMode
  Saturation : Saturate  UpperLimit=2000  LowerLimit=1000
  Saturation1 : Saturate  UpperLimit=1  LowerLimit=0
  Saturation10 : Saturate  UpperLimit=deg2rad(50)  LowerLimit=-deg2rad(50)
  Saturation2 : Saturate  UpperLimit=1  LowerLimit=0
  Saturation3 : Saturate  UpperLimit=1  LowerLimit=-1
  Saturation4 : Saturate  UpperLimit=1  LowerLimit=-1
  Saturation5 : Saturate  UpperLimit=1  LowerLimit=-1
  Saturation6 : Saturate  UpperLimit=1  LowerLimit=0
  Saturation7 : Saturate  UpperLimit=deg2rad(20)  LowerLimit=-deg2rad(20)
  Saturation8 : Saturate  UpperLimit=2  LowerLimit=-2
  Saturation9 : Saturate  UpperLimit=deg2rad(20)  LowerLimit=-deg2rad(20)
  Selector : Selector  InputPortWidth=3  IndexOptions=Index vector (dialog)  Indices=[3 2 1]  OutputSizes=1
  Selector1 : Selector  InputPortWidth=3  IndexOptions=Index vector (dialog)  Indices=3  OutputSizes=1
  Sqrt : Sqrt
  Square : Math  Operator=square
  Subsystem : Subsystem
  Sum{,1..7} (8 alike) : Sum  Inputs=|+-
  Switch{,1..11} (12 alike) : Switch  Threshold=1  SaturateOnIntegerOverflow=off  InputSameDT=off
  Transpose : Math  Operator=transpose
  Motor_PWM_cmd : Outport
  wires:
  Sum/1 -> PID Controller/1
  Copter_States/1 -> Bus Selector/1, Bus Selector1/1
  Bus Selector/1 -> [euler_angles_feedback_rad], Demux/1  "<euler_rad>"
  Bus Selector/2 -> Demux1/1  "<angular_vel_b_rads>"
  Demux/1 -> [roll_angle_feedback_rad]
  Demux/2 -> [pitch_angle_feedback_rad]
  Demux/3 -> [yaw_angle_feedback_rad]
  Demux1/1 -> [p_feedback_rads]
  Demux1/2 -> [q_feedback_rads]
  Demux1/3 -> [r_feedback_rads]
  Sum1/1 -> PID Controller1/1
  Sum2/1 -> PID Controller2/1
  [r_feedback_rads] -> Sum2/2
  PID Controller3/1 -> Sum/1
  Sum3/1 -> PID Controller3/1
  Sum4/1 -> PID Controller4/1
  [pitch_angle_feedback_rad] -> Sum4/2
  Bus Selector1/1 -> Demux2/1  "<pos_e_m>"
  Bus Selector1/2 -> Demux4/1  "<vel_e_ms>"
  Bus Selector1/3 -> [accel_be_feedback_mss]  "<accel_be_mss>"
  Demux4/3 -> [vel_z_e_feedback_ms]
  Demux2/3 -> [pos_z_e_feedback_m]
  Sum6/1 -> PID Controller6/1
  Sum7/1 -> PID Controller7/1
  [pos_z_e_feedback_m] -> Gain1/1
  Constant3/1 -> Sum7/1
  Gain/1 -> Sum6/2
  Gain1/1 -> Sum7/2
  Gain2/1 -> Sum5/2
  Gain3/1 -> Add1/1
  Constant4/1 -> Add1/2
  Add1/1 -> Saturation/1
  [vel_z_e_feedback_ms] -> Gain/1
  [roll_cmd] -> Saturation7/1
  Constant5/1 -> Add2/1
  Constant6/1 -> Add2/2
  Gain4/1 -> Add3/1
  Add2/1 -> Add4/2, Gain5/1
  Gain5/1 -> Square/1
  Square/1 -> Add3/2
  Add3/1 -> Sqrt/1
  Sqrt/1 -> Add4/1
  Add4/1 -> Divide/1
  Constant7/1 -> Divide/2
  Divide/1 -> Saturation6/1
  Saturation3/1 -> Subsystem/3(tau_yaw)
  Saturation4/1 -> Subsystem/2(tau_pitch)
  Saturation5/1 -> Subsystem/1(tau_roll)
  Saturation2/1 -> Subsystem/4(totalThrust)
  Keyboard 1/1 -> [Key]
  Keyboard 1/2 -> [KeybIn]
  [Key] -> Equal/2
  Constant8/1 -> Equal/1
  Equal1/1 -> [positive_roll]
  Constant9/1 -> Equal1/1
  [Key] -> Equal1/2
  [Key] -> Equal2/2
  Constant10/1 -> Equal2/1
  Equal3/1 -> [positive_pitch]
  Constant11/1 -> Equal3/1
  [Key] -> Equal3/2
  [positive_yaw] -> AND/1
  [KeybIn] -> AND/2
  Discrete-Time Integrator/1 -> Degrees to Radians/1
  Add5/1 -> Discrete-Time Integrator/1
  Equal2/1 -> [negative_pitch]
  Equal/1 -> [negative_roll]
  AND/1 -> OR/1, Switch/2
  Constant2/1 -> Switch/1
  Constant12/1 -> Switch/3
  Constant13/1 -> Switch1/3
  AND2/1 -> Switch1/2, OR/2
  [KeybIn] -> AND2/2
  [negative_yaw] -> AND2/1
  Constant14/1 -> Switch1/1
  Switch/1 -> Add5/1
  Switch1/1 -> Add5/2
  Degrees to Radians/1 -> [yaw_cmd]
  [pitch_cmd] -> Saturation9/1
  Constant15/1 -> Switch2/1
  Constant16/1 -> Switch2/3
  Switch2/1 -> Discrete-Time Integrator1/1
  Discrete-Time Integrator1/1 -> Equal4/1
  Constant19/1 -> Equal4/2
  Equal4/1 -> Discrete-Time Integrator/2
  OR/1 -> Discrete-Time Integrator1/2, Switch2/2
  OR1/1 -> Switch5/2, Discrete-Time Integrator3/2
  Equal5/1 -> Discrete-Time Integrator2/2
  Constant23/1 -> Equal5/2
  Discrete-Time Integrator3/1 -> Equal5/1
  Switch5/1 -> Discrete-Time Integrator3/1
  Constant22/1 -> Switch5/3
  Constant21/1 -> Switch5/1
  Degrees to Radians1/1 -> [pitch_cmd]
  Switch4/1 -> Add6/2
  Switch3/1 -> Add6/1
  Constant20/1 -> Switch4/1
  [negative_pitch] -> AND3/1
  [KeybIn] -> AND3/2
  AND3/1 -> OR1/2, Switch4/2
  Constant18/1 -> Switch4/3
  Constant17/1 -> Switch3/3
  Constant24/1 -> Switch3/1
  AND1/1 -> Switch3/2, OR1/1
  Add6/1 -> Discrete-Time Integrator2/1
  Discrete-Time Integrator2/1 -> Degrees to Radians1/1
  [KeybIn] -> AND1/2
  [positive_pitch] -> AND1/1
  [up] -> AND4/1
  [KeybIn] -> AND4/2
  Add7/1 -> Discrete-Time Integrator4/1
  AND4/1 -> OR2/1, Switch6/2
  Constant31/1 -> Switch6/1
  Constant25/1 -> Switch6/3
  Constant26/1 -> Switch7/3
  AND5/1 -> Switch7/2, OR2/2
  [KeybIn] -> AND5/2
  [down] -> AND5/1
  Constant27/1 -> Switch7/1
  Switch6/1 -> Add7/1
  Switch7/1 -> Add7/2
  Constant28/1 -> Switch8/1
  Constant29/1 -> Switch8/3
  Switch8/1 -> Discrete-Time Integrator5/1
  Discrete-Time Integrator5/1 -> Equal6/1
  Constant30/1 -> Equal6/2
  Equal6/1 -> Discrete-Time Integrator4/2
  OR2/1 -> Discrete-Time Integrator5/2, Switch8/2
  OR3/1 -> Switch11/2, Discrete-Time Integrator7/2
  Equal7/1 -> Discrete-Time Integrator6/2
  Constant37/1 -> Equal7/2
  Discrete-Time Integrator7/1 -> Equal7/1
  Switch11/1 -> Discrete-Time Integrator7/1
  Constant36/1 -> Switch11/3
  Constant35/1 -> Switch11/1
  Degrees to Radians3/1 -> [roll_cmd]
  Switch10/1 -> Add8/2
  Switch9/1 -> Add8/1
  Constant34/1 -> Switch10/1
  [negative_roll] -> AND7/1
  [KeybIn] -> AND7/2
  AND7/1 -> OR3/2, Switch10/2
  Constant33/1 -> Switch10/3
  Constant32/1 -> Switch9/3
  Constant38/1 -> Switch9/1
  AND6/1 -> Switch9/2, OR3/1
  Add8/1 -> Discrete-Time Integrator6/1
  Discrete-Time Integrator6/1 -> Degrees to Radians3/1
  [KeybIn] -> AND6/2
  [positive_roll] -> AND6/1
  Equal8/1 -> [positive_yaw]
  [Key] -> Equal9/2
  Constant40/1 -> Equal9/1
  Equal9/1 -> [negative_yaw]
  Constant39/1 -> Equal8/1
  [Key] -> Equal8/2
  [Key] -> Equal10/2
  Constant41/1 -> Equal10/1
  Equal11/1 -> [up]
  Constant42/1 -> Equal11/1
  [Key] -> Equal11/2
  Equal10/1 -> [down]
  Discrete-Time Integrator4/1 -> [thrst_cmd]
  [thrst_cmd] -> Saturation8/1
  [yaw_cmd] -> Saturation10/1
  [p_feedback_rads] -> Sum/2
  PID Controller4/1 -> Sum1/1
  [roll_angle_feedback_rad] -> Sum3/2
  Saturation1/1 -> Gain3/1
  [q_feedback_rads] -> Sum1/2
  Subsystem/1(thrusts_refout) -> Saturation1/1
  Saturation8/1 -> Sum6/1
  PID Controller/1 -> Saturation5/1
  PID Controller1/1 -> Saturation4/1
  PID Controller2/1 -> Saturation3/1
  Saturation/1 -> Motor_PWM_cmd/1
  PID Controller5/1 -> Saturation2/1
  PID Controller6/1 -> Sum5/1
  Sum5/1 -> PID Controller5/1
  Constant/1 -> Add/2
  [euler_angles_feedback_rad] -> Selector/1
  Selector/1 -> Rotation Angles to Direction Cosine Matrix/1
  Rotation Angles to Direction Cosine Matrix/1 -> Transpose/1
  Transpose/1 -> Matrix Multiply/1
  [accel_be_feedback_mss] -> Matrix Multiply/2
  Matrix Multiply/1 -> Selector1/1
  Selector1/1 -> Add/1
  Add/1 -> Gain2/1
  Saturation7/1 -> Sum3/1
  Saturation9/1 -> Sum4/1
  Saturation10/1 -> Sum2/1

== system Quad_F450_Model/Copter Properties ==
  Arm_1 : Subsystem
  Arm_2 : Subsystem
  Arm_3 : Subsystem
  Arm_4 : Subsystem
  Bus Creator : BusCreator  Inputs=5
  Subsystem : Subsystem
  Copter : Outport
  wires:
  Arm_1/1(Arm_1) -> [Arm_1]
  Subsystem/1(Copter_Frame) -> [Copter_Frame]
  [Copter_Frame] -> Bus Creator/5  "Frame"
  [Arm_4] -> Bus Creator/4  "Arm_4"
  [Arm_3] -> Bus Creator/3  "Arm_3"
  [Arm_1] -> Bus Creator/1  "Arm_1"
  [Arm_2] -> Bus Creator/2  "Arm_2"
  Bus Creator/1 -> Copter/1
  Arm_4/1(Arm_4) -> [Arm_4]
  Arm_3/1(Arm_3) -> [Arm_3]
  Arm_2/1(Arm_2) -> [Arm_2]

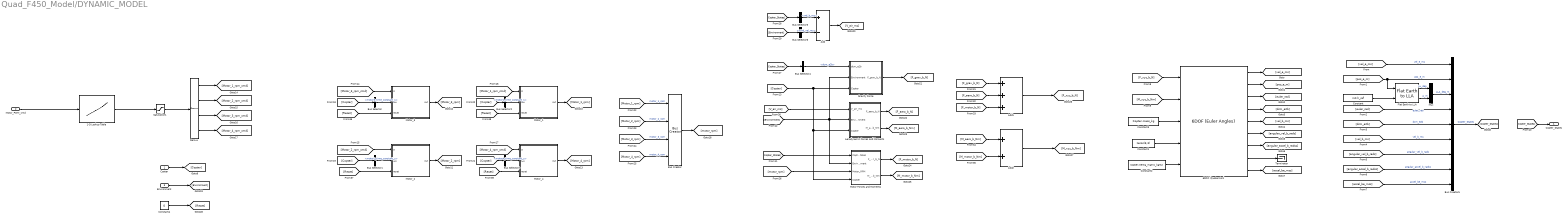
== system Quad_F450_Model/DYNAMIC_MODEL ==
  Copter : Inport
  Motor_PWM_cmd : Inport  Port=2
  Environment : Inport  Port=3
  1-D Lookup Table : Lookup_n-D  NumberOfTableDimensions=1  BreakpointsForDimension1=flipud(motor_data.PWMThrottleSignals)  Table=flipud(motor_data.RotationSpeedrpm)  ExtrapMethod=Clip  UseLastTableValue=on  ApplyFullPrecisionForLinearInterpolation=on  InternalRulePriority=Speed  RndMeth=Simplest
  6DOF (Quaternion) : shared6dof/6DOF (Euler Angles)  units=Metric (MKS)  mtype=Custom Variable  rep=Quaternion  xme_0=init.pos_e_m  Vm_0=init.vel_b_ms  eul_0=init.euler_rad  pm_0=init.ang_vel_rads  mass_0=Copter.mass_kg  mass_e=0.5  mass_f=2.0  inertia=Copter.inertia_matrix_kgm2  inertia_e=eye(3)  inertia_f=2*eye(3)  k_quat=1.0  vre_flag=off  abi_flag=on  aMode=0  xme_statename=''  Vm_statename=''  eul_statename=''  quat_statename=''  pm_statename=''  mass_statename=''
      settings: LibrarySourceBlock=aerolib6dof2/6DOF (Quaternion)
  Add : Sum  Inputs=+-
  Add1 : Sum  Inputs=3
  Add2 : Sum  Inputs=2
  Aerodynamic Forces and Moments : Subsystem
  Bus Creator : BusCreator  Inputs=4
  Bus Creator5 : BusCreator  Inputs=9
  Bus Selector : BusSelector  OutputSignals=Arm_3.motor3_time_constant_s
  Bus Selector1 : BusSelector  OutputSignals=Arm_2.motor2_time_constant_s
  Bus Selector2 : BusSelector  OutputSignals=Arm_1.motor1_time_constant_s
  Bus Selector3 : BusSelector  OutputSignals=Arm_4.motor4_time_constant_s
  Bus Selector4 : BusSelector  OutputSignals=dcm_e2b
  Bus Selector5 : BusSelector  OutputSignals=vel_b_ms
  Bus Selector6 : BusSelector  OutputSignals=wind_vel_ms
  Constant : Constant  Value=init.h_ref
  Constant1 : Constant  Value=zeros(3,3)
  Constant2 : Constant  Value=Copter.inertia_matrix_kgm2
  Constant3 : Constant  Value=Copter.mass_kg
  Constant4 : Constant  Value=0
  Demux : Demux
  Flat Earth to LLA : aerolibtransform2/Flat Earth to LLA  units=Metric (MKS)  ptype=Earth (WGS84)  F=1/298.257223563  R=6378137  refPosPort=off  LL0=init.pos_LLA_deg(1:2)  psi=0
  "Gravity Force " : Subsystem
  Motor Forces and Moments : Subsystem
  Motor_1 : Subsystem
  Motor_2 : Subsystem
  Motor_3 : Subsystem
  Motor_4 : Subsystem
  Mux : Mux  Inputs=2
  Saturation1 : Saturate  UpperLimit=10000  LowerLimit=100
  Terminator : Terminator
  Copter_States : Outport
  wires:
  6DOF (Quaternion)/1 -> [vel_e_ms]
  6DOF (Quaternion)/3 -> [euler_rad]
  6DOF (Quaternion)/4 -> [dcm_e2b]
  6DOF (Quaternion)/5 -> [vel_b_ms]
  6DOF (Quaternion)/6 -> [angular_vel_b_rads]
  6DOF (Quaternion)/7 -> [angular_accel_b_radss]
  6DOF (Quaternion)/8 -> Terminator/1
  6DOF (Quaternion)/9 -> [accel_be_mss]
  6DOF (Quaternion)/2 -> [pos_e_m]
  [dcm_e2b] -> Bus Creator5/5  "dcm_e2b"
  [accel_be_mss] -> Bus Creator5/9  "accel_be_mss"
  Bus Creator5/1 -> [Copter_States]  "Copter_States"
  [angular_accel_b_radss] -> Bus Creator5/8  "angular_accel_b_radss"
  [angular_vel_b_rads] -> Bus Creator5/7  "angular_vel_b_rads"
  [pos_e_m] -> Flat Earth to LLA/1, Bus Creator5/2  "pos_e_m"
  [vel_e_ms] -> Bus Creator5/1  "vel_e_ms"
  [euler_rad] -> Bus Creator5/4  "euler_rad"
  [vel_b_ms] -> Bus Creator5/6  "vel_b_ms"
  Constant/1 -> Flat Earth to LLA/2
  Flat Earth to LLA/1 -> Mux/1  "LL_deg"
  Mux/1 -> Bus Creator5/3  "LLA_deg_m"
  Flat Earth to LLA/2 -> Mux/2  "A_m"
  [F_xyz_b_N] -> 6DOF (Quaternion)/1
  [M_xyz_b_Nm] -> 6DOF (Quaternion)/2
  [Copter_States] -> Copter_States/1
  Constant1/1 -> 6DOF (Quaternion)/4
  Constant2/1 -> 6DOF (Quaternion)/5
  Constant3/1 -> 6DOF (Quaternion)/3
  [Copter] -> Motor Forces and Moments/4(Copter), Aerodynamic Forces and Moments/3(Copter), "Gravity Force "/3(Copter)
  Copter/1 -> [Copter]
  Motor_1/1(out) -> [Motor_1_rpm]
  Motor_2/1(out) -> [Motor_2_rpm]
  Motor_3/1(out) -> [Motor_3_rpm]
  Motor_4/1(out) -> [Motor_4_rpm]
  [Motor_3_rpm_cmd] -> Motor_3/1(in)
  [Motor_2_rpm_cmd] -> Motor_2/1(in)
  [Motor_1_rpm_cmd] -> Motor_1/1(in)
  [Motor_4_rpm_cmd] -> Motor_4/1(in)
  [Copter] -> Bus Selector/1
  Bus Selector/1 -> Motor_3/2(tau)  "<motor3_time_constant_s>"
  [Copter] -> Bus Selector1/1
  Bus Selector1/1 -> Motor_2/2(tau)  "<motor2_time_constant_s>"
  [Copter] -> Bus Selector2/1
  Bus Selector2/1 -> Motor_1/2(tau)  "<motor1_time_constant_s>"
  [Copter] -> Bus Selector3/1
  Bus Selector3/1 -> Motor_4/2(tau)  "<motor4_time_constant_s>"
  Demux/2 -> [Motor_2_rpm_cmd]
  Demux/1 -> [Motor_1_rpm_cmd]
  Demux/3 -> [Motor_3_rpm_cmd]
  Demux/4 -> [Motor_4_rpm_cmd]
  [Motor_4_rpm] -> Bus Creator/4  "motor_4_rpm"
  [Motor_3_rpm] -> Bus Creator/3  "motor_3_rpm"
  [Motor_2_rpm] -> Bus Creator/2  "motor_2_rpm"
  [Motor_1_rpm] -> Bus Creator/1  "motor_1_rpm"
  Bus Creator/1 -> [motor_rpm]
  [motor_rpm] -> Motor Forces and Moments/3(Motor_RPM)
  [Environment] -> "Gravity Force "/2(Environment), Motor Forces and Moments/2(Environment), Aerodynamic Forces and Moments/2(Environment)
  Environment/1 -> [Environment]
  [Copter_States] -> Motor Forces and Moments/1(Copter_States)
  [Copter_States] -> Bus Selector4/1
  Bus Selector4/1 -> "Gravity Force "/1(dcm_e2b)  "<dcm_e2b>"
  [Copter_States] -> Bus Selector5/1
  [Environment] -> Bus Selector6/1
  Bus Selector5/1 -> Add/1  "<vel_b_ms>"
  Bus Selector6/1 -> Add/2  "<wind_vel_ms>"
  Add/1 -> [V_air_ms]
  [V_air_ms] -> Aerodynamic Forces and Moments/1(V_air_ms)
  Aerodynamic Forces and Moments/1(F_aero_b_N) -> [F_aero_b_N]
  Aerodynamic Forces and Moments/2(M_aero_b_Nm) -> [M_aero_b_Nm]
  [F_motor_b_N] -> Add1/3
  [F_aero_b_N] -> Add1/2
  [F_grav_b_N] -> Add1/1
  [M_aero_b_Nm] -> Add2/1
  [M_motor_b_Nm] -> Add2/2
  Add2/1 -> [M_xyz_b_Nm]
  [Reset] -> Motor_3/3(reset)
  [Reset] -> Motor_2/3(reset)
  [Reset] -> Motor_1/3(reset)
  [Reset] -> Motor_4/3(reset)
  Constant4/1 -> [Reset]
  Add1/1 -> [F_xyz_b_N]
  "Gravity Force "/1(F_grav_b_N) -> [F_grav_b_N]
  Motor_PWM_cmd/1 -> 1-D Lookup Table/1
  1-D Lookup Table/1 -> Saturation1/1
  Saturation1/1 -> Demux/1
  Motor Forces and Moments/1(F_motor_b_N) -> [F_motor_b_N]
  Motor Forces and Moments/2(M_motor_b_Nm) -> [M_motor_b_Nm]

== system Quad_F450_Model/ENVIRONMENT ==
  Copter_States : Inport
  Bus Creator : BusCreator  Inputs=3
  Bus Creator1 : BusCreator  Inputs=4
  Bus Selector : BusSelector  OutputSignals=LLA_deg_m
  COESA Atmosphere Model : aerolibatmos2/COESA Atmosphere Model  units=Metric (MKS)  spec=1976 COESA-extended U.S. Standard Atmosphere  model=Profile  profile_var=High temperature  profile_percent=1%  profile_alt=5 km (16404 ft)  envelope_var=High temperature  envelope_percent=1%  action=Warning
  Selector : Selector  InputPortWidth=3  IndexOptions=Index vector (dialog)  Indices=3  OutputSizes=1
  Subsystem : Subsystem
  "WGS84 Gravity Model  " : GravityWGS84
  Environment : Outport  VectorParamsAs1DForOutWhenUnconnected=off
  wires:
  Bus Creator/1 -> Environment/1
  COESA Atmosphere Model/4 -> Bus Creator1/4  "air_density_kgm3"
  COESA Atmosphere Model/2 -> Bus Creator1/2  "speed_sound_ms"
  Bus Creator1/1 -> Bus Creator/2  "Atmosphere_Prop"
  COESA Atmosphere Model/3 -> Bus Creator1/3  "pressure_Pa"
  COESA Atmosphere Model/1 -> Bus Creator1/1  "air_temp_K"
  "WGS84 Gravity Model  "/1 -> Bus Creator/1  "gravity_e_mss"
  Subsystem/1(wind_vel_ms) -> Bus Creator/3  "wind_vel_ms"
  Copter_States/1 -> Bus Selector/1
  Bus Selector/1 -> Selector/1, "WGS84 Gravity Model  "/1  "<LLA_deg_m>"
  Selector/1 -> COESA Atmosphere Model/1

== system Quad_F450_Model/Controller/Subsystem ==
  tau_roll : Inport
  tau_pitch : Inport  Port=2
  tau_yaw : Inport  Port=3
  totalThrust : Inport  Port=4
  Constant : Constant  Value=Controller.Control_Allocation
  Mux2 : Mux
  Product : Product  Multiplication=Matrix(*)  RndMeth=Zero
  thrusts_refout : Outport  VectorParamsAs1DForOutWhenUnconnected=off
  wires:
  Product/1 -> thrusts_refout/1
  Mux2/1 -> Product/2
  totalThrust/1 -> Mux2/1
  Constant/1 -> Product/1
  tau_yaw/1 -> Mux2/4
  tau_roll/1 -> Mux2/2
  tau_pitch/1 -> Mux2/3
